simulink model "cruise_control_model2"  (R2018a)
settings: Solver=VariableStepAuto  StartTime=0.0  StopTime=10.0  RelTol=1e-3
settings Model: Creator=3  LastModifiedBy=3

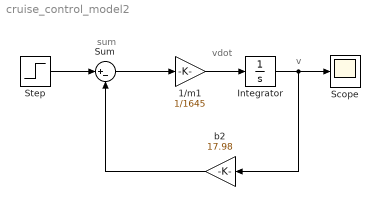
== system cruise_control_model2 ==
  note: v
  note: sum
  note: vdot
  1/m1 : Gain  Gain=1/1645
  Integrator : Integrator
  Scope : Scope
  Step : Step  Time=0  After=26.8  SampleTime=0
  Sum : Sum  Inputs=|+-
  b2 : Gain  Gain=17.98
  wires:
  Integrator/1 -> Scope/1, b2/1
  Step/1 -> Sum/1
  1/m1/1 -> Integrator/1
  Sum/1 -> 1/m1/1
  b2/1 -> Sum/2
